simulink subsystem "Subsystem"  (R2021a)
settings: Solver=VariableStepAuto  StartTime=0.0  StopTime=10.0  RelTol=1e-3
undefined symbols (not defined in the file or in its folder): T
settings Model: Creator=Faaor  LastModifiedBy=Faaor

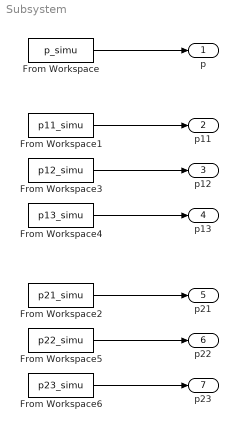
== system Subsystem ==
  From Workspace : FromWorkspace  VariableName=p_simu  SampleTime=T
  From Workspace1 : FromWorkspace  VariableName=p11_simu  SampleTime=T
  From Workspace2 : FromWorkspace  VariableName=p21_simu  SampleTime=T
  From Workspace3 : FromWorkspace  VariableName=p12_simu  SampleTime=T
  From Workspace4 : FromWorkspace  VariableName=p13_simu  SampleTime=T
  From Workspace5 : FromWorkspace  VariableName=p22_simu  SampleTime=T
  From Workspace6 : FromWorkspace  VariableName=p23_simu  SampleTime=T
  p : Outport
  p11 : Outport  Port=2
  p12 : Outport  Port=3
  p13 : Outport  Port=4
  p21 : Outport  Port=5
  p22 : Outport  Port=6
  p23 : Outport  Port=7
  wires:
  From Workspace1/1 -> p11/1
  From Workspace4/1 -> p13/1
  From Workspace3/1 -> p12/1
  From Workspace/1 -> p/1
  From Workspace6/1 -> p23/1
  From Workspace5/1 -> p22/1
  From Workspace2/1 -> p21/1
